simulink model "myDCMotorControl"  (R2019a)
settings: Solver=FixedStepAuto  StartTime=0.0  StopTime=inf  RelTol=1e-3  EnableMultiTasking=on
values from neighbouring files (symbols this model uses):
  PWMcmdMono = [-1 -0.95 -0.9 -0.85 -0.8 -0.75 -0.7 -0.65 -0.6 -0.55 -0.5 -0.45 ... (39 elements, 1x39)]    [motorResponse.mat]
  speedMono = [-5044.36055317 -4862.51266484 -4633.2869083 -4350.79106811 -4105.01838263 -3802.89419016 -3514.14649909 -3245.90349257 -2990.70453206 -2680.14555765 -2434.1528594 -2138.37828068 ... (39 elements, 1x39)]    [motorResponse.mat]
undefined symbols (not defined in the file or in its folder): Ts
libraries: mkrmotorcarrierlib x2
settings Model: SimulationMode=external  ExtModeTrigDuration=2  Creator=mugiwarra  LastModifiedBy=mugiwarra
settings OptimizationCC: EnhancedBackFolding=on  PassReuseOutputArgsAs=Individual arguments  MaxStackSize=64  OptimizeBlockOrder=speed  DifferentSizesBufferReuse=on  OptimizationCustomize=off
settings DebuggingCC: ParameterTunabilityLossMsg=error
settings HardwareCC: ProdBitPerPointer=32  ProdBitPerSizeT=32  ProdBitPerPtrDiffT=32  ProdLargestAtomicInteger=Long  ProdLargestAtomicFloat=Double  ProdWordSize=32  ProdHWDeviceType=ARM Compatible->ARM Cortex  UseEmbeddedCoderFeatures=off  UseSimulinkCoderFeatures=off
settings SFSimCC: MATLABDynamicMemAlloc=off
settings RTWCC: SystemTargetFile=ert.tlc  HardwareBoard=Arduino MKR1000  TLCOptions=-aInlineSetEventsForThisBaseRateFcn=TLC_FALSE -aSuppressMultiTaskScheduler=TLC_FALSE -aRateBasedStepFcn=1  TemplateMakefile=ert_default_tmf  GenerateReport=on  Toolchain=Arduino ARM  BuildConfiguration=Faster Runs  IncludeHyperlinkInReport=on  LaunchReport=on  GenerateTraceInfo=on  GenerateTraceReport=on  GenerateTraceReportSl=on  GenerateTraceReportSf=on  GenerateTraceReportEml=on
settings CodeAppCC: ForceParamTrailComments=on  IgnoreCustomStorageClasses=off  OperatorAnnotations=on  SimulinkDataObjDesc=on  SFDataObjDesc=on  InsertBlockDesc=on
settings ERTTargetCC: SupportContinuousTime=on  SupportNonInlinedSFcns=on  SupportVariableSizeSignals=on  ExtModeStaticAllocSize=8192

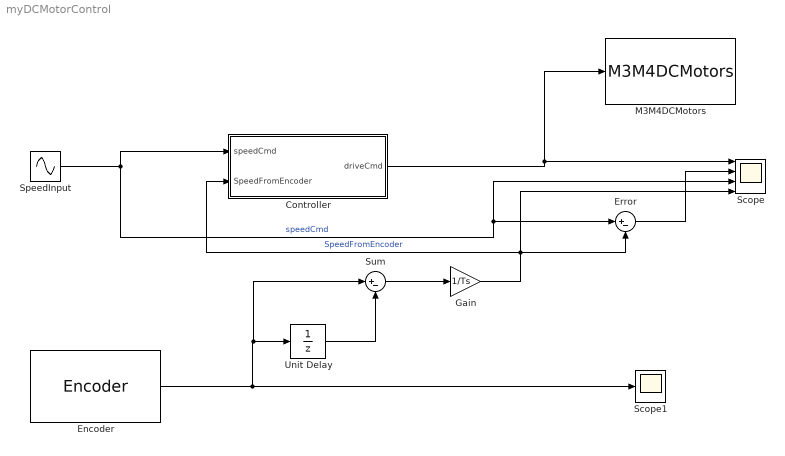
== system myDCMotorControl ==
  Controller : Subsystem
  Encoder : mkrmotorcarrierlib/Encoder  SlaveAddress=uint8(102)  blockPlatform=ARDUINO  Encoder=1  ShowSpeed=off  ResetOption=off  SampleTime=0.1
      settings: SourceProductName=Simulink Support Package for Arduino Hardware  SourceProductBaseCode=ARDUINO
  Error : Sum  Inputs=|+-
  Gain : Gain  Gain=1/Ts
  M3M4DCMotors : mkrmotorcarrierlib/M3M4DCMotors  MotorNumber=M3
      settings: SourceProductName=Simulink Support Package for Arduino Hardware  SourceProductBaseCode=ARDUINO
  Scope : Scope  NumInputPorts=4
  Scope1 : Scope
  "SpeedInput " : Sin  Amplitude=6000  SampleTime=Ts
  Sum : Sum  Inputs=|+-
  Unit Delay : UnitDelay  SampleTime=-1  HasFrameUpgradeWarning=on
  wires:
  "SpeedInput "/1 -> Error/1, Scope/3, Controller/1(speedCmd)  "speedCmd"
  Controller/1(driveCmd) -> M3M4DCMotors/1, Scope/1
  Encoder/1 -> Sum/1, Unit Delay/1, Scope1/1
  Sum/1 -> Gain/1
  Unit Delay/1 -> Sum/2
  Gain/1 -> Controller/2(SpeedFromEncoder), Error/2, Scope/4  "SpeedFromEncoder"
  Error/1 -> Scope/2

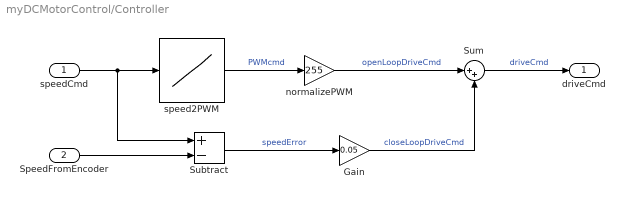
== system myDCMotorControl/Controller ==
  speedCmd : Inport
  SpeedFromEncoder : Inport  Port=2
  Gain : Gain  Gain=0.05
  Subtract : Sum  Inputs=+-
  Sum : Sum  Inputs=|++
  normalizePWM : Gain  Gain=255
  speed2PWM : Lookup_n-D  NumberOfTableDimensions=1  BreakpointsForDimension1=speedMono  Table=PWMcmdMono  InternalRulePriority=Speed  RndMeth=Simplest  InputSameDT=on
  driveCmd : Outport
  wires:
  speed2PWM/1 -> normalizePWM/1  "PWMcmd"
  speedCmd/1 -> Subtract/1, speed2PWM/1
  SpeedFromEncoder/1 -> Subtract/2
  Subtract/1 -> Gain/1  "speedError"
  Gain/1 -> Sum/2  "closeLoopDriveCmd"
  normalizePWM/1 -> Sum/1  "openLoopDriveCmd"
  Sum/1 -> driveCmd/1  "driveCmd"
